simulink model "homework601"  (R2019b)
settings: Solver=VariableStepAuto  StartTime=0.0  StopTime=10.0  RelTol=1e-3
settings Model: Creator=路西法  LastModifiedBy=Lenovo
settings DataIOCC: ReturnWorkspaceOutputs=off
settings DebuggingCC: ArithmeticOperatorsInVariantConditions=warning
settings SFSimCC: SimUseLocalCustomCode=off  CustomCodeUndefinedFunction=UseInterfaceOnly
settings RTWCC: RTWUseLocalCustomCode=off

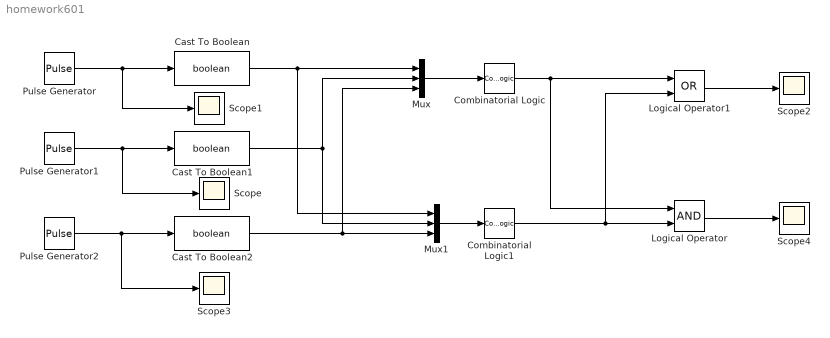
== system homework601 ==
  Cast To Boolean : DataTypeConversion  OutDataTypeStr=boolean
  Cast To Boolean1 : DataTypeConversion  OutDataTypeStr=boolean
  Cast To Boolean2 : DataTypeConversion  OutDataTypeStr=boolean
  Combinatorial Logic : CombinatorialLogic  TruthTable=[1;1;1;1;1;1;0;1]
  Combinatorial Logic1 : CombinatorialLogic  TruthTable=[1;0;0;0;0;0;0;1]
  Logical Operator : Logic  AllPortsSameDT=off  OutDataTypeStr=boolean
  Logical Operator1 : Logic  Operator=OR  AllPortsSameDT=off  OutDataTypeStr=boolean
  Mux : Mux  Inputs=3
  Mux1 : Mux  Inputs=3
  Pulse Generator : DiscretePulseGenerator  PhaseDelay=1  SampleTime=4
  Pulse Generator1 : DiscretePulseGenerator  PhaseDelay=1  SampleTime=2
  Pulse Generator2 : DiscretePulseGenerator  PhaseDelay=1
  Scope{,1..4} (5 alike) : Scope
  wires:
  Pulse Generator1/1 -> Scope/1, Cast To Boolean1/1
  Pulse Generator/1 -> Scope1/1, Cast To Boolean/1
  Pulse Generator2/1 -> Scope3/1, Cast To Boolean2/1
  Mux/1 -> Combinatorial Logic/1
  Mux1/1 -> Combinatorial Logic1/1
  Combinatorial Logic/1 -> Logical Operator/1, Logical Operator1/1
  Combinatorial Logic1/1 -> Logical Operator1/2, Logical Operator/2
  Cast To Boolean/1 -> Mux1/1, Mux/1
  Cast To Boolean1/1 -> Mux1/2, Mux/2
  Cast To Boolean2/1 -> Mux1/3, Mux/3
  Logical Operator/1 -> Scope4/1
  Logical Operator1/1 -> Scope2/1
